simulink model "ques2"  (R2021a)
settings: Solver=VariableStepAuto  StartTime=0.0  StopTime=100  RelTol=1e-3
model workspace (MAT data in the model file):
  b = Simulink.Parameter
  b.Value = 1000
  b.DataType = 'auto'
  b.Dimensions = [1 1]
  k1 = Simulink.Parameter
  k1.Value = 36000
  k1.DataType = 'auto'
  k1.Dimensions = [1 1]
  k2 = Simulink.Parameter
  k2.Value = 204030
  k2.DataType = 'auto'
  k2.Dimensions = [1 1]
  m1 = Simulink.Parameter
  m1.Value = 600
  m1.DataType = 'auto'
  m1.Dimensions = [1 1]
  m2 = Simulink.Parameter
  m2.Value = 80
  m2.DataType = 'auto'
  m2.Dimensions = [1 1]
undefined symbols (not defined in the file): sigbuilder_block
settings Model: Creator=AVM  LastModifiedBy=AVM

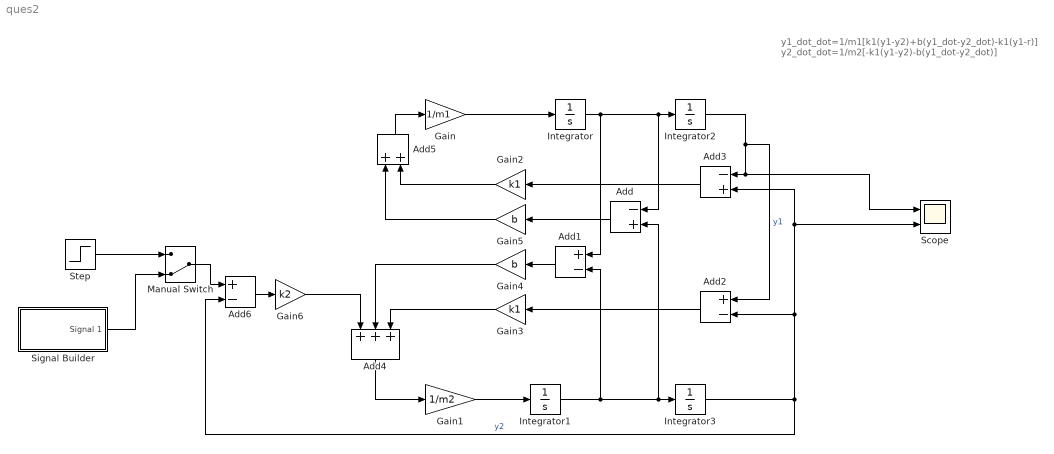
== system ques2 ==
  note: y1_dot_dot=1/m1[k1(y1-y2)+b(y1_dot-y2_dot)-k1(y1-r)]
      | y2_dot_dot=1/m2[-k1(y1-y2)-b(y1_dot-y2_dot)]
  Add : Sum  Inputs=-+
  Add1 : Sum  Inputs=+-
  Add2 : Sum  Inputs=+-
  Add3 : Sum  Inputs=-+
  Add4 : Sum  Inputs=+++
  Add5 : Sum
  Add6 : Sum  Inputs=+-
  Gain : Gain  Gain=1/m1
  Gain1 : Gain  Gain=1/m2
  Gain2 : Gain  Gain=k1
  Gain3 : Gain  Gain=k1
  Gain4 : Gain  Gain=b
  Gain5 : Gain  Gain=b
  Gain6 : Gain  Gain=k2
  Integrator{,1..3} (4 alike) : Integrator
  Manual Switch : ManualSwitch  CurrentSetting=0
  Scope : Scope  NumInputPorts=2
  Signal Builder : Subsystem  Tag=STV Subsys  LoadFcn=sigbuilder_block('load');  StartFcn=sigbuilder_block('start');  StopFcn=sigbuilder_block('stop');  ClipboardFcn=sigbuilder_block('clipboard');  mask(Sigbuilder block){tuvar=[0:10]}
      mask help: Simulink:masks:SigbuilderBlock_MD
      mask init:
      | if ~strcmp(get_param(bdroot(gcbh),'SimulationStatus'),'stopped') tuvar = sigbuilder_block('maskInit'); end
      settings: CopyFcn=sigbuilder_block('copy');  DeleteFcn=sigbuilder_block('delete');  ModelCloseFcn=sigbuilder_block('modelClose');  PreSaveFcn=sigbuilder_block('preSave');  PauseFcn=sigbuilder_block('pause');  ContinueFcn=sigbuilder_block('continue');  NameChangeFcn=sigbuilder_block('namechange');  OpenFcn=sigbuilder_block('open',[437.6 153.75 550.4 359.25 ]);  CloseFcn=sigbuilder_block('close');
      mask Display: plot(0, 0, 100, 100,[2, 2, 32, 32, 2], [68, 8, 8, 68, 68],[32, 2], [38, 38], [32, 19, 2],[53, 60, 44], [32, 17, 17, 2],[16, 16, 31, 31]);txt = getActiveGroup(gcbh);text(2, 100, txt,'verticalAlignment', 'top');
  Step : Step  SampleTime=0
  wires:
  Add1/1 -> Gain4/1
  Gain5/1 -> Add5/1
  Add2/1 -> Gain3/1
  Integrator2/1 -> Scope/1, Add3/1, Add2/1  "y1"
  Gain4/1 -> Add4/2
  Integrator1/1 -> Add1/2, Add/2, Integrator3/1
  Add3/1 -> Gain2/1
  Gain/1 -> Integrator/1
  Integrator/1 -> Add1/1, Add/1, Integrator2/1
  Gain6/1 -> Add4/1
  Gain2/1 -> Add5/2
  Add5/1 -> Gain/1
  Add6/1 -> Gain6/1
  Integrator3/1 -> Add6/2, Scope/2, Add3/2, Add2/2  "y2"
  Add/1 -> Gain5/1
  Gain3/1 -> Add4/3
  Manual Switch/1 -> Add6/1
  Add4/1 -> Gain1/1
  Gain1/1 -> Integrator1/1
  Step/1 -> Manual Switch/1
  Signal Builder/1(Signal 1) -> Manual Switch/2

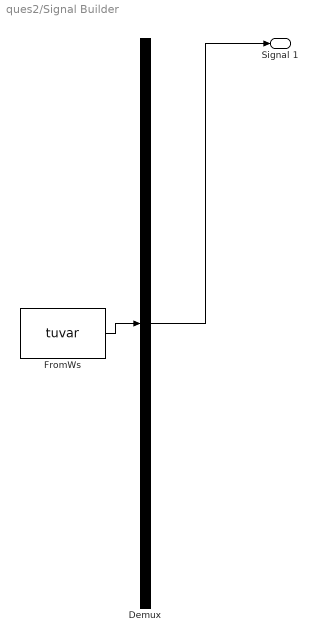
== system ques2/Signal Builder ==
  Demux : Demux  Tag=STV Demux  Outputs=1
      settings: DisplayOption=none
  FromWs : FromWorkspace  Tag=STV FromWs  VariableName=tuvar  OutputAfterFinalValue=Holding final value
      SigBuilderData=|
      | common.afterFinalStr = 'Hold final value'
      | common.sampleTime = '0'
      | dataSet.timeRange = [0 10]
      | dataSet.name = 'Group 1'
      | sbobj.Groups.Name = 'Group 1'
      | sbobj.Groups.Signals.Name = 'Signal 1'
      | sbobj.Groups.Signals.XData = [0 0.54 1.56 2.34 2.82 4 4 4.65 5.35 6 6.6 7.52 8.62 9.48 10]
      | sbobj.Groups.Signals.YData = [0 0.03 0.324797687861 0.57 0.73 1.03 1.02 1.13 1.16 1.12 1.01 0.69 0.36 0.08 -0.01]
      | sbobj.Groups.TimeRange = [0 10]
  Signal 1 : Outport  Tag=STV Outport
  wires:
  Demux/1 -> Signal 1/1
  FromWs/1 -> Demux/1
